simulink model "celcius_to_fahrenheit"  (R2020b)
settings: Solver=ode45  StartTime=0.0  StopTime=10.0  RelTol=1e-3  EnableMultiTasking=on
settings Model: Creator=USER  LastModifiedBy=USER
settings DataIOCC: LimitDataPoints=on  SaveFormat=Array  ReturnWorkspaceOutputs=off
settings OptimizationCC: LifeSpan=inf
settings DebuggingCC: SFUnexpectedBacktrackingDiag=warning  SFNoUnconditionalDefaultTransitionDiag=warning  SFExecutionAtInitializationDiag=none  ArithmeticOperatorsInVariantConditions=warning
settings HardwareCC: ProdBitPerPointer=32  ProdBitPerSizeT=32  ProdBitPerPtrDiffT=32  ProdLargestAtomicFloat=None  ProdIntDivRoundTo=Undefined  ProdEndianess=Unspecified  ProdWordSize=32  ProdHWDeviceType=32-bit Generic
settings ModelReferenceCC: PropagateSignalLabelsOutOfModel=off
settings SFSimCC: SimUseLocalCustomCode=off  CustomCodeUndefinedFunction=UseInterfaceOnly
settings RTWCC: RTWUseLocalCustomCode=off
settings CodeAppCC: StateflowObjectComments=on
settings GRTTargetCC: TargetLangStandard=C89/C90 (ANSI)
settings ConfigComp: CovMetricSettings=dw  CovSaveCumulativeToWorkspaceVar=on  CovSaveSingleToWorkspaceVar=on  CovExternalEMLEnable=off

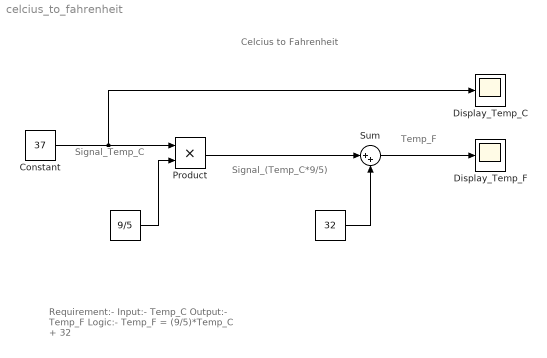
== system celcius_to_fahrenheit ==
  note: Requirement:-
      |
      | Input:- Temp_C
      | Output:- Temp_F
      | Logic:- Temp_F = (9/5)*Temp_C + 32
  note: Temp_F
  note: Signal_(Temp_C*9/5)
  note: Signal_Temp_C
  note: Celcius to Fahrenheit
  " " : Constant  Value=9/5
  " " : Constant  Value=32
  Constant : Constant  Value=37
  Display_Temp_C : Scope
  Display_Temp_F : Scope
  Product : Product
  Sum : Sum  Inputs=|++
  wires:
  Constant/1 -> Display_Temp_C/1, Product/1
  " "/1 -> Product/2
  Product/1 -> Sum/1
  " "/1 -> Sum/2
  Sum/1 -> Display_Temp_F/1
